simulink model "Electrical_System_2018b_obfs"  (R2019b)
settings: Solver=VariableStepAuto  StartTime=0.0  StopTime=5  RelTol=1e-3  AbsTol=1e-3  EnableMultiTasking=on
InitFcn:
  | Steady_State_Initialisation;
StopFcn:
  | %sscexplore(simlog);
  | %Logging
undefined symbols (not defined in the file): abrlhklxvp, aexgmhuedq, afmfmjnutg, afpphrjpnc, ahuxbyvruc, alarvljztt, amxnyqmnuw, aodrlwvqie, aolhmuplyq, aqpmguuqkg, auesgwirzl, aurophlnng, awamelrhru, ayfhvxflxn, azxkacuhqc, babszerikg, bawhdqanwq, bevoqecvei, bltjvqbchx, bmqsuewujl, bsmyqjfgnf, btvjbsmnve, bywgxqeadw, bziaduxaer, bzmcmdqocb, bzsvyvetat, ccsjnrbsih, cdvenygxwh, cedkrnslhx, cjheorclzs, cjrdshrtqx, ckhavyhcza, ckxewznhlz, cmrcgyiplk, conenicnws, cqkejbgjnn, csfnuwymhe, cunupkhwbh, cwzfvzuxxh, dcadmadufn, dcfponivnv, ddtrqjrhjn, dfhoxvkqas, dfrhtcwpne, dfvomcagjv, djijwylxea, dnmeqksrrm, dnzewbdkaa, dsqcykyxav, dtswwlttmm, ecumpidjtv, edegaywrct, ejjjsmnejc, eknqnehjdz, emvdetzouf, esxbqkbahr, etnkkbreiq, eunoiiiirw, ewewcuedir, fatkfxdhtc ... (+386)
libraries: fl_lib x802, ee_lib x362, fl_ps_legacy_lib x160, nesl_utility x85
(part 1 of 26)
settings Model: Creator=u617417  LastModifiedBy=u617417
settings SolverCC: AutoScaleAbsTol=off
settings DataIOCC: LimitDataPoints=on  MaxDataPoints=10000  ReturnWorkspaceOutputs=off
settings OptimizationCC: LifeSpan=inf
settings DebuggingCC: AllowSymbolicDim=off  SFUnexpectedBacktrackingDiag=warning  SFNoUnconditionalDefaultTransitionDiag=warning  SFExecutionAtInitializationDiag=none  ArithmeticOperatorsInVariantConditions=warning
settings SFSimCC: SimUseLocalCustomCode=off  CustomCodeUndefinedFunction=UseInterfaceOnly
settings RTWCC: RTWUseLocalCustomCode=off
settings CodeAppCC: StateflowObjectComments=on
settings GRTTargetCC: TargetLangStandard=C89/C90 (ANSI)  GeneratePreprocessorConditionals=Disable all
settings ConfigComp: CovMetricSettings=dw  CovHtmlReporting=on  CovSaveCumulativeToWorkspaceVar=on  CovSaveSingleToWorkspaceVar=on  CovExternalEMLEnable=off  CovSFcnEnable=off
settings SimscapeCC: SimscapeLogType=all  SimscapeLogDataHistory=10000

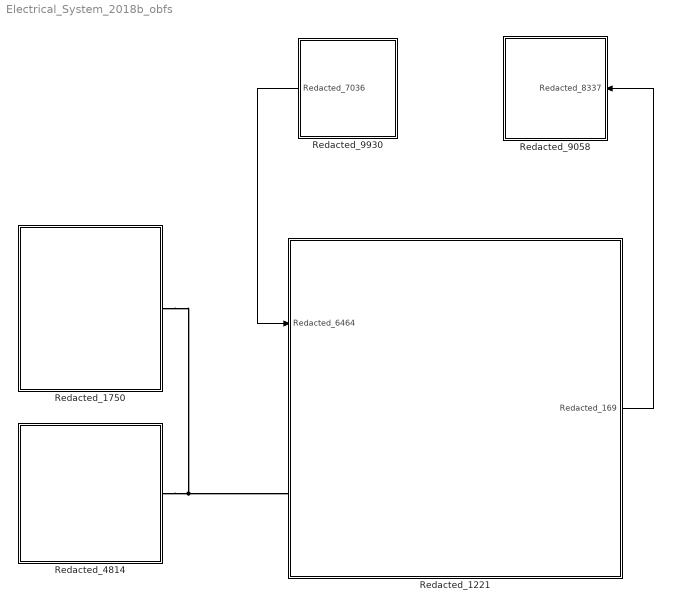
== system Electrical_System_2018b_obfs ==
  Redacted_1221 : Subsystem
  Redacted_1750 : Subsystem
  Redacted_4814 : Subsystem
  Redacted_9058 : Subsystem
  Redacted_9930 : Subsystem
  wires:
  Redacted_9930/1(Redacted_7036) -> Redacted_1221/1(Redacted_6464)
  Redacted_1221/1(Redacted_169) -> Redacted_9058/1(Redacted_8337)
  connections:
  Redacted_4814/RConn1 -- Redacted_1750/LConn1 -- Redacted_1221/LConn1

== system Electrical_System_2018b_obfs/Redacted_1221 ==
  Redacted_6464 : Inport
  Redacted_124 : BusCreator  Inputs=2
  Redacted_1290 : SimscapeBus  HierarchyStrings=Redacted_9542;Redacted_7385
  Redacted_346 : Subsystem
  Redacted_3922 : BusSelector  OutputSignals=Redacted1000,Redacted100
  Redacted_7523 : Subsystem
  Redacted_7580 : BusCreator  Inputs=2
  Redacted_7996 : Subsystem
  Redacted_7064 : PMIOPort  Side=Left
  Redacted_169 : Outport
  wires:
  Redacted_6464/1 -> Redacted_3922/1, Redacted_7996/1(Redacted_8884)
  Redacted_3922/2 -> Redacted_7523/1(Redacted_6806)  "<Redacted100>"
  Redacted_7996/1(Redacted_414) -> Redacted_7580/1
  Redacted_3922/1 -> Redacted_346/1(Redacted_388)  "<Redacted1000>"
  Redacted_124/1 -> Redacted_7580/2
  Redacted_7580/1 -> Redacted_169/1
  Redacted_346/1(Redacted_1936) -> Redacted_124/1
  Redacted_7523/1(Redacted_1117) -> Redacted_124/2
  connections:
  Redacted_7996/LConn1 -- Redacted_1290/RConn1 -- Redacted_7064/RConn1
  Redacted_7523/LConn1 -- Redacted_1290/LConn2
  Redacted_1290/LConn1 -- Redacted_346/LConn1

== system Electrical_System_2018b_obfs/Redacted_1750 ==
  Redacted_1744 : SimscapeBus  HierarchyStrings=Redacted_3580;Redacted_2679;Redacted_1356;Redacted_4546;Redacted_2723;Redacted_3875;Redacted_702;Redacted_7645;Redacted_1338;Redacted_3379;Redacted_7168;Redacted_7354;Redacted_1728;Redacted_6589;Redacted_3064;Redacted_7149;Redacted_7529;Redacted_4383;Redacted_4107;Redacted_3568;Redacted_6624;Redacted_6947;Redacted_2339;Redacted_4294;Redacted_5075;Redacted_5111;Redacted_7066;Redacted_1531;Redacted_7675;Redacted_9811;Redacted_5065;Redacted_4812;Redacted_9201;Redacted_6197;Redacted_8441;Redacted_5922;Redacted_720;Redacted_3478
  Redacted_1805 : SimscapeBus  HierarchyStrings=Redacted_9383;Redacted_6662
  Redacted_1925 : Subsystem  VariantControlMode=Label  Variant=on  VariantControl=Variant1  LabelModeActiveChoice=Choice
  Redacted_2252 : Subsystem  VariantControlMode=Label  Variant=on  VariantControl=Variant1  LabelModeActiveChoice=Choice
  Redacted_3116 : Subsystem  VariantControlMode=Label  Variant=on  VariantControl=Variant1  LabelModeActiveChoice=Variant1
  Redacted_342 : SimscapeBus  HierarchyStrings=Redacted_4753;Redacted_7074;Redacted_4542;Redacted_1072;Redacted_6392;Redacted_7262;Redacted_2302;Redacted_3799;Redacted_313;Redacted_3360;Redacted_9805;Redacted_7349;Redacted_7947;Redacted_2722;Redacted_9575;Redacted_197;Redacted_61;Redacted_5963;Redacted_4867;Redacted_743;Redacted_7386;Redacted_3425;Redacted_4607;Redacted_2034;Redacted_2575;Redacted_353;Redacted_234;Redacted_6669;Redacted_5669;Redacted_4890;Redacted_9806;Redacted_6181;Redacted_8668;Redacted_4306;Redacted_593;Redacted_8425;Redacted_5908;Redacted_8012;Redacted_3708;Redacted_3632;Redacted_250;Redacted_5917;Redacted_5879;Redacted_6182;Redacted_5408;Redacted_9552;Redacted_4609;Redacted_5680;Redacted_7438;Redacted_5551
  Redacted_3629 : Subsystem  VariantControlMode=Label  Variant=on  VariantControl=Variant1  LabelModeActiveChoice=Choice
  Redacted_3745 : SimscapeBus  HierarchyStrings=Redacted_1096;Redacted_3567
  Redacted_3761 : SimscapeBus  HierarchyStrings=Redacted_780;Redacted_28
  Redacted_393 : Subsystem  VariantControlMode=Label  Variant=on  VariantControl=Variant1  LabelModeActiveChoice=Choice
  Redacted_418 : Subsystem  VariantControlMode=Label  Variant=on  VariantControl=Variant1  LabelModeActiveChoice=Choice
  Redacted_4904 : nesl_utility/Solver Configuration  PhysicalDomain=network_engine_domain  SubClassName=solver  LeftPortType=input  RightPortType=generic  Tones=[]  Harmonics=[]  SimulateNoise=off  Profile=off  UseLocalSampling=off  EnableSwitchedLinearOptims=on  FrequencyDomain=off  UseCCode=off  RelTol=0.001  AbsTol=1e-06  MinStep=1e-09  ToWorkspace=off  RevertToSquareIcSolve=off  NumHomotopyIterations=100  PhasorMode=off  PhasorModeNumHarmonics=1  DoDC=on  ResidualTolerance=1e-09  UseLocalSolver=off  LocalSolverChoice=NE_BACKWARD_EULER_ADVANCER  LocalSolverSampleTime=0.001  DoFixedCost=off  MaxNonlinIter=3  MaxModeIter=2  LinearAlgebra=auto  EquationFormulation=NE_TIME_EF  DelaysMemoryBudget=1024  AutomaticFiltering=on  FilteringTimeConstant=0.001  PartitionStorageMethod=AS_NEEDED  PartitionMemoryBudget=1024  PartitionMethod=FAST
  Redacted_4947 : Subsystem
  Redacted_5338 : SimscapeBus  HierarchyStrings=Redacted_4565;Redacted_3565;Redacted_3754;Redacted_3229;Redacted_1463;Redacted_2424;Redacted_1593;Redacted_6398;Redacted_2122;Redacted_5759;Redacted_1474;Redacted_4040;Redacted_2796;Redacted_8639;Redacted_7131;Redacted_6318;Redacted_7850;Redacted_3335;Redacted_4313;Redacted_1636;Redacted_1179;Redacted_2852;Redacted_8529;Redacted_9943;Redacted_3136;Redacted_6249;Redacted_7332;Redacted_6303;Redacted_8216;Redacted_7695;Redacted_8718;Redacted_3072;Redacted_1178;Redacted_1890;Redacted_6383;Redacted_2665;Redacted_4351;Redacted_4540;Redacted_8937;Redacted_7401;Redacted_7023;Redacted_5287;Redacted_2225;Redacted_314;Redacted_4153;Redacted_6133;Redacted_6666;Redacted_1276;Redacted_2787;Redacted_6122
  Redacted_5639 : Subsystem
  Redacted_5682 : Subsystem  VariantControlMode=Label  Variant=on  VariantControl=Variant1  LabelModeActiveChoice=Choice
  Redacted_7456 : Subsystem  VariantControlMode=Label  Variant=on  VariantControl=Variant1  LabelModeActiveChoice=Variant1
  Redacted_7650 : Subsystem  VariantControlMode=Label  Variant=on  VariantControl=Variant1  LabelModeActiveChoice=Choice
  Redacted_8299 : Subsystem  VariantControlMode=Label  Variant=on  VariantControl=Variant1  LabelModeActiveChoice=Choice
  Redacted_8526 : SimscapeBus  HierarchyStrings=Redacted_5196;Redacted_4738;Redacted_9034;Redacted_8939;Redacted_5097;Redacted_5335;Redacted_8921;Redacted_9654;Redacted_7688;Redacted_4574;Redacted_6489;Redacted_3669;Redacted_1425;Redacted_9271;Redacted_8750;Redacted_5309;Redacted_2108;Redacted_3147;Redacted_7076;Redacted_768;Redacted_3463;Redacted_9121;Redacted_3800;Redacted_3593;Redacted_7030;Redacted_595;Redacted_9929;Redacted_1003;Redacted_3651;Redacted_3255;Redacted_1785;Redacted_2177;Redacted_6543;Redacted_5208;Redacted_247;Redacted_4433;Redacted_4655;Redacted_3962
  Redacted_8712 : Subsystem  VariantControlMode=Label  Variant=on  VariantControl=Variant1  LabelModeActiveChoice=Choice
  Redacted_1626 : PMIOPort  Side=Left
  connections:
  Redacted_418/LConn1 -- Redacted_342/LConn27
  Redacted_1744/LConn5 -- Redacted_4947/LConn5
  Redacted_418/LConn4 -- Redacted_342/LConn30
  Redacted_418/LConn3 -- Redacted_342/LConn29
  Redacted_1744/LConn1 -- Redacted_4947/LConn1
  Redacted_4947/LConn4 -- Redacted_1744/LConn4
  Redacted_1744/LConn3 -- Redacted_4947/LConn3
  Redacted_4947/LConn6 -- Redacted_1744/LConn6
  Redacted_418/LConn2 -- Redacted_342/LConn28
  Redacted_7650/LConn1 -- Redacted_342/LConn31
  Redacted_7650/LConn2 -- Redacted_342/LConn32
  Redacted_7650/LConn3 -- Redacted_342/LConn33
  Redacted_7650/LConn4 -- Redacted_342/LConn34
  Redacted_7650/LConn5 -- Redacted_342/LConn35
  Redacted_7650/LConn6 -- Redacted_342/LConn36
  Redacted_7650/LConn7 -- Redacted_342/LConn37
  Redacted_7650/LConn8 -- Redacted_342/LConn38
  Redacted_1925/LConn1 -- Redacted_342/LConn39
  Redacted_1925/LConn2 -- Redacted_342/LConn40
  Redacted_1925/LConn3 -- Redacted_342/LConn41
  Redacted_1925/LConn4 -- Redacted_342/LConn42
  Redacted_1925/LConn5 -- Redacted_342/LConn43
  Redacted_1925/LConn6 -- Redacted_342/LConn44
  Redacted_5338/LConn27 -- Redacted_393/LConn1
  Redacted_5338/LConn28 -- Redacted_393/LConn2
  Redacted_5338/LConn29 -- Redacted_393/LConn3
  Redacted_5338/LConn30 -- Redacted_393/LConn4
  Redacted_5338/LConn39 -- Redacted_8299/LConn1
  Redacted_5338/LConn40 -- Redacted_8299/LConn2
  Redacted_5338/LConn41 -- Redacted_8299/LConn3
  Redacted_5338/LConn42 -- Redacted_8299/LConn4
  Redacted_5338/LConn43 -- Redacted_8299/LConn5
  Redacted_5338/LConn44 -- Redacted_8299/LConn6
  Redacted_5338/LConn31 -- Redacted_3629/LConn1
  Redacted_5338/LConn32 -- Redacted_3629/LConn2
  Redacted_5338/LConn33 -- Redacted_3629/LConn3
  Redacted_5338/LConn34 -- Redacted_3629/LConn4
  Redacted_5338/LConn35 -- Redacted_3629/LConn5
  Redacted_5338/LConn36 -- Redacted_3629/LConn6
  Redacted_5338/LConn37 -- Redacted_3629/LConn7
  Redacted_5338/LConn38 -- Redacted_3629/LConn8
  Redacted_4904/RConn1 -- Redacted_5338/LConn47 -- Redacted_5682/RConn4
  Redacted_5682/LConn1 -- Redacted_342/LConn50
  Redacted_5682/LConn2 -- Redacted_342/LConn49
  Redacted_5682/LConn3 -- Redacted_342/LConn48
  Redacted_5682/LConn4 -- Redacted_342/LConn47
  Redacted_5338/LConn50 -- Redacted_5682/RConn1
  Redacted_5338/LConn49 -- Redacted_5682/RConn2
  Redacted_5338/LConn48 -- Redacted_5682/RConn3
  Redacted_4947/LConn2 -- Redacted_1744/LConn2
  Redacted_1744/LConn7 -- Redacted_4947/LConn7
  Redacted_4947/LConn8 -- Redacted_1744/LConn8
  Redacted_3745/RConn1 -- Redacted_1626/RConn1
  Redacted_1744/LConn9 -- Redacted_4947/LConn9
  Redacted_1744/LConn10 -- Redacted_4947/LConn10
  Redacted_1744/LConn14 -- Redacted_4947/LConn14
  Redacted_1744/LConn13 -- Redacted_4947/LConn13
  Redacted_1744/LConn12 -- Redacted_4947/LConn12
  Redacted_4947/LConn11 -- Redacted_1744/LConn11
  Redacted_1744/RConn1 -- Redacted_3761/LConn2
  Redacted_3761/LConn1 -- Redacted_342/RConn1
  Redacted_1805/LConn1 -- Redacted_5338/RConn1
  Redacted_3761/RConn1 -- Redacted_3745/LConn2
  Redacted_1805/RConn1 -- Redacted_3745/LConn1
  Redacted_4947/LConn15 -- Redacted_1744/LConn15
  Redacted_4947/LConn16 -- Redacted_1744/LConn16
  Redacted_4947/LConn17 -- Redacted_1744/LConn17
  Redacted_4947/LConn18 -- Redacted_1744/LConn18
  Redacted_4947/LConn19 -- Redacted_1744/LConn19
  Redacted_4947/LConn20 -- Redacted_1744/LConn20
  Redacted_4947/LConn21 -- Redacted_1744/LConn21
  Redacted_4947/LConn22 -- Redacted_1744/LConn22
  Redacted_4947/LConn23 -- Redacted_1744/LConn23
  Redacted_4947/LConn24 -- Redacted_1744/LConn24
  Redacted_4947/LConn25 -- Redacted_1744/LConn25
  Redacted_4947/LConn26 -- Redacted_1744/LConn26
  Redacted_4947/LConn27 -- Redacted_1744/LConn27
  Redacted_4947/LConn28 -- Redacted_1744/LConn28
  Redacted_4947/LConn29 -- Redacted_1744/LConn29
  Redacted_4947/LConn30 -- Redacted_1744/LConn30
  Redacted_2252/LConn1 -- Redacted_342/LConn1
  Redacted_2252/LConn2 -- Redacted_342/LConn2
  Redacted_2252/LConn3 -- Redacted_342/LConn3
  Redacted_2252/LConn4 -- Redacted_342/LConn4
  Redacted_2252/LConn5 -- Redacted_342/LConn5
  Redacted_2252/LConn6 -- Redacted_342/LConn6
  Redacted_2252/LConn7 -- Redacted_342/LConn7
  Redacted_2252/LConn8 -- Redacted_342/LConn8
  Redacted_2252/LConn9 -- Redacted_342/LConn9
  Redacted_2252/LConn10 -- Redacted_342/LConn10
  Redacted_2252/LConn11 -- Redacted_342/LConn11
  Redacted_2252/LConn12 -- Redacted_342/LConn12
  Redacted_2252/LConn13 -- Redacted_342/LConn13
  Redacted_2252/LConn14 -- Redacted_342/LConn14
  Redacted_2252/LConn15 -- Redacted_342/LConn15
  Redacted_2252/LConn16 -- Redacted_342/LConn16
  Redacted_2252/LConn17 -- Redacted_342/LConn17
  Redacted_2252/LConn18 -- Redacted_342/LConn18
  Redacted_2252/LConn19 -- Redacted_342/LConn19
  Redacted_2252/LConn20 -- Redacted_342/LConn20
  Redacted_2252/LConn21 -- Redacted_342/LConn21
  Redacted_2252/LConn22 -- Redacted_342/LConn22
  Redacted_2252/LConn23 -- Redacted_342/LConn23
  Redacted_2252/LConn24 -- Redacted_342/LConn24
  Redacted_2252/LConn25 -- Redacted_342/LConn25
  Redacted_2252/LConn26 -- Redacted_342/LConn26
  Redacted_4947/LConn31 -- Redacted_1744/LConn31
  Redacted_4947/LConn33 -- Redacted_1744/LConn33
  Redacted_4947/LConn35 -- Redacted_1744/LConn35
  Redacted_4947/LConn36 -- Redacted_1744/LConn36
  Redacted_4947/LConn37 -- Redacted_1744/LConn37
  Redacted_4947/LConn38 -- Redacted_1744/LConn38
  Redacted_4947/LConn34 -- Redacted_1744/LConn34
  Redacted_4947/LConn32 -- Redacted_1744/LConn32
  Redacted_8712/LConn1 -- Redacted_5338/LConn1
  Redacted_8712/LConn2 -- Redacted_5338/LConn2
  Redacted_8712/LConn3 -- Redacted_5338/LConn3
  Redacted_8712/LConn4 -- Redacted_5338/LConn4
  Redacted_8712/LConn5 -- Redacted_5338/LConn5
  Redacted_8712/LConn6 -- Redacted_5338/LConn6
  Redacted_8712/LConn7 -- Redacted_5338/LConn7
  Redacted_8712/LConn8 -- Redacted_5338/LConn8
  Redacted_8712/LConn9 -- Redacted_5338/LConn9
  Redacted_8712/LConn10 -- Redacted_5338/LConn10
  Redacted_8712/LConn11 -- Redacted_5338/LConn11
  Redacted_8712/LConn12 -- Redacted_5338/LConn12
  Redacted_8712/LConn13 -- Redacted_5338/LConn13
  Redacted_8712/LConn14 -- Redacted_5338/LConn14
  Redacted_8712/LConn15 -- Redacted_5338/LConn15
  Redacted_8712/LConn16 -- Redacted_5338/LConn16
  Redacted_8712/LConn17 -- Redacted_5338/LConn17
  Redacted_8712/LConn18 -- Redacted_5338/LConn18
  Redacted_8712/LConn19 -- Redacted_5338/LConn19
  Redacted_8712/LConn20 -- Redacted_5338/LConn20
  Redacted_8712/LConn21 -- Redacted_5338/LConn21
  Redacted_8712/LConn22 -- Redacted_5338/LConn22
  Redacted_8712/LConn23 -- Redacted_5338/LConn23
  Redacted_8712/LConn24 -- Redacted_5338/LConn24
  Redacted_8712/LConn25 -- Redacted_5338/LConn25
  Redacted_8712/LConn26 -- Redacted_5338/LConn26
  Redacted_5639/LConn32 -- Redacted_8526/LConn32
  Redacted_5639/LConn34 -- Redacted_8526/LConn34
  Redacted_5639/LConn37 -- Redacted_8526/LConn37
  Redacted_5639/LConn35 -- Redacted_8526/LConn35
  Redacted_5639/LConn33 -- Redacted_8526/LConn33
  Redacted_5639/LConn31 -- Redacted_8526/LConn31
  Redacted_5639/LConn30 -- Redacted_8526/LConn30
  Redacted_5639/LConn29 -- Redacted_8526/LConn29
  Redacted_5639/LConn28 -- Redacted_8526/LConn28
  Redacted_5639/LConn36 -- Redacted_8526/LConn36
  Redacted_5639/LConn27 -- Redacted_8526/LConn27
  Redacted_5639/LConn25 -- Redacted_8526/LConn25
  Redacted_5639/LConn24 -- Redacted_8526/LConn24
  Redacted_5639/LConn23 -- Redacted_8526/LConn23
  Redacted_5639/LConn22 -- Redacted_8526/LConn22
  Redacted_5639/LConn21 -- Redacted_8526/LConn21
  Redacted_5639/LConn20 -- Redacted_8526/LConn20
  Redacted_5639/LConn19 -- Redacted_8526/LConn19
  Redacted_5639/LConn18 -- Redacted_8526/LConn18
  Redacted_5639/LConn17 -- Redacted_8526/LConn17
  Redacted_5639/LConn16 -- Redacted_8526/LConn16
  Redacted_5639/LConn26 -- Redacted_8526/LConn26
  Redacted_5639/LConn38 -- Redacted_8526/LConn38
  Redacted_5639/LConn15 -- Redacted_8526/LConn15
  Redacted_5639/LConn11 -- Redacted_8526/LConn11
  Redacted_8526/LConn12 -- Redacted_5639/LConn12
  Redacted_8526/LConn13 -- Redacted_5639/LConn13
  Redacted_8526/LConn10 -- Redacted_5639/LConn10
  Redacted_8526/LConn9 -- Redacted_5639/LConn9
  Redacted_5639/LConn8 -- Redacted_8526/LConn8
  Redacted_5639/LConn6 -- Redacted_8526/LConn6
  Redacted_8526/LConn7 -- Redacted_5639/LConn7
  Redacted_8526/LConn3 -- Redacted_5639/LConn3
  Redacted_5639/LConn4 -- Redacted_8526/LConn4
  Redacted_8526/LConn1 -- Redacted_5639/LConn1
  Redacted_8526/LConn14 -- Redacted_5639/LConn14
  Redacted_8526/LConn5 -- Redacted_5639/LConn5
  Redacted_5639/LConn2 -- Redacted_8526/LConn2
  Redacted_8526/RConn1 -- Redacted_1805/LConn2
  Redacted_3116/LConn1 -- Redacted_342/LConn45
  Redacted_3116/LConn2 -- Redacted_342/LConn46
  Redacted_7456/LConn1 -- Redacted_5338/LConn45
  Redacted_7456/LConn2 -- Redacted_5338/LConn46

== system Electrical_System_2018b_obfs/Redacted_4814 ==
  Redacted_1188 : SimscapeBus  HierarchyStrings=Redacted_5170;Redacted_3456
  Redacted_1224 : SimscapeBus  HierarchyStrings=Redacted_5417;Redacted_5050
  Redacted_1389 : SimscapeBus  HierarchyStrings=Redacted_4470;Redacted_2451
  Redacted_3297 : Subsystem  VariantControlMode=Label  Variant=on  VariantControl=Variant1  LabelModeActiveChoice=Choice
  Redacted_3902 : SimscapeBus  HierarchyStrings=Redacted_1356;Redacted_9036
  Redacted_3928 : Subsystem  VariantControlMode=Label  Variant=on  VariantControl=Variant1  LabelModeActiveChoice=Choice
  Redacted_7520 : SimscapeBus  HierarchyStrings=Redacted_3429;Redacted_1098
  Redacted_8098 : SimscapeBus  HierarchyStrings=Redacted_379;Redacted_2486
  Redacted_8799 : SimscapeBus  HierarchyStrings=Redacted_3276;Redacted_5658
  Redacted_9979 : PMIOPort  Side=Right
  connections:
  Redacted_3297/RConn1 -- Redacted_8098/LConn1
  Redacted_1188/RConn1 -- Redacted_9979/RConn1
  Redacted_7520/RConn1 -- Redacted_1188/LConn2
  Redacted_8098/LConn2 -- Redacted_3297/RConn2
  Redacted_8799/LConn2 -- Redacted_3297/RConn4
  Redacted_8799/LConn1 -- Redacted_3297/RConn3
  Redacted_1389/LConn2 -- Redacted_8799/RConn1
  Redacted_1389/LConn1 -- Redacted_8098/RConn1
  Redacted_1389/RConn1 -- Redacted_1188/LConn1
  Redacted_7520/LConn1 -- Redacted_3902/RConn1
  Redacted_7520/LConn2 -- Redacted_1224/RConn1
  Redacted_3902/LConn1 -- Redacted_3928/RConn1
  Redacted_3902/LConn2 -- Redacted_3928/RConn2
  Redacted_3928/RConn3 -- Redacted_1224/LConn1
  Redacted_3928/RConn4 -- Redacted_1224/LConn2

== system Electrical_System_2018b_obfs/Redacted_9058 ==
  Redacted_8337 : Inport
  Redacted_8297 : Terminator
  wires:
  Redacted_8337/1 -> Redacted_8297/1

== system Electrical_System_2018b_obfs/Redacted_9930 ==
  Redacted_2381 : BusCreator  Inputs=30
  Redacted_3896 : Subsystem  VariantControlMode=Label  Variant=on  VariantControl=Variant1  LabelModeActiveChoice=Variant1
  Redacted_4112 : BusCreator  Inputs=30
  Redacted_4814 : Subsystem  VariantControlMode=Label  Variant=on  VariantControl=Variant1  LabelModeActiveChoice=Variant1
  Redacted_6072 : BusCreator  Inputs=2
  Redacted_7036 : Outport
  wires:
  Redacted_6072/1 -> Redacted_7036/1
  Redacted_4112/1 -> Redacted_6072/2  "Redacted1000"
  Redacted_2381/1 -> Redacted_6072/1  "Redacted100"
  Redacted_3896/1(Redacted_644) -> Redacted_2381/1
  Redacted_3896/2(Redacted_2723) -> Redacted_2381/2
  Redacted_3896/3(Redacted_8075) -> Redacted_2381/3
  Redacted_3896/4(Redacted_4126) -> Redacted_2381/4
  Redacted_3896/5(Redacted_7964) -> Redacted_2381/5
  Redacted_3896/6(Redacted_8682) -> Redacted_2381/6
  Redacted_3896/7(Redacted_6320) -> Redacted_2381/7
  Redacted_3896/8(Redacted_340) -> Redacted_2381/8
  Redacted_3896/9(Redacted_2756) -> Redacted_2381/9
  Redacted_3896/10(Redacted_3273) -> Redacted_2381/10
  Redacted_3896/11(Redacted_4657) -> Redacted_2381/11
  Redacted_3896/12(Redacted_3395) -> Redacted_2381/12
  Redacted_3896/13(Redacted_9977) -> Redacted_2381/13
  Redacted_3896/14(Redacted_2599) -> Redacted_2381/14
  Redacted_3896/15(Redacted_1407) -> Redacted_2381/15
  Redacted_3896/16(Redacted_9412) -> Redacted_2381/16
  Redacted_3896/17(Redacted_123) -> Redacted_2381/17
  Redacted_3896/18(Redacted_8209) -> Redacted_2381/18
  Redacted_3896/19(Redacted_531) -> Redacted_2381/19
  Redacted_3896/20(Redacted_6389) -> Redacted_2381/20
  Redacted_3896/21(Redacted_6836) -> Redacted_2381/21
  Redacted_3896/22(Redacted_5007) -> Redacted_2381/22
  Redacted_3896/23(Redacted_6497) -> Redacted_2381/23
  Redacted_3896/24(Redacted_9632) -> Redacted_2381/24
  Redacted_3896/25(Redacted_2902) -> Redacted_2381/25
  Redacted_3896/26(Redacted_2695) -> Redacted_2381/26
  Redacted_3896/27(Redacted_8396) -> Redacted_2381/27
  Redacted_3896/28(Redacted_9164) -> Redacted_2381/28
  Redacted_3896/29(Redacted_9075) -> Redacted_2381/29
  Redacted_3896/30(Redacted_6090) -> Redacted_2381/30
  Redacted_4814/1(Redacted_6479) -> Redacted_4112/1
  Redacted_4814/2(Redacted_3532) -> Redacted_4112/2
  Redacted_4814/3(Redacted_6579) -> Redacted_4112/3
  Redacted_4814/4(Redacted_5091) -> Redacted_4112/4
  Redacted_4814/5(Redacted_5066) -> Redacted_4112/5
  Redacted_4814/6(Redacted_2648) -> Redacted_4112/6
  Redacted_4814/7(Redacted_3799) -> Redacted_4112/7
  Redacted_4814/8(Redacted_988) -> Redacted_4112/8
  Redacted_4814/9(Redacted_4741) -> Redacted_4112/9
  Redacted_4814/10(Redacted_474) -> Redacted_4112/10
  Redacted_4814/11(Redacted_4041) -> Redacted_4112/11
  Redacted_4814/12(Redacted_9998) -> Redacted_4112/12
  Redacted_4814/13(Redacted_2742) -> Redacted_4112/13
  Redacted_4814/14(Redacted_5781) -> Redacted_4112/14
  Redacted_4814/15(Redacted_125) -> Redacted_4112/15
  Redacted_4814/16(Redacted_4308) -> Redacted_4112/16
  Redacted_4814/17(Redacted_8077) -> Redacted_4112/17
  Redacted_4814/18(Redacted_7701) -> Redacted_4112/18
  Redacted_4814/19(Redacted_8967) -> Redacted_4112/19
  Redacted_4814/20(Redacted_8464) -> Redacted_4112/20
  Redacted_4814/21(Redacted_1093) -> Redacted_4112/21
  Redacted_4814/22(Redacted_1950) -> Redacted_4112/22
  Redacted_4814/23(Redacted_1167) -> Redacted_4112/23
  Redacted_4814/24(Redacted_3969) -> Redacted_4112/24
  Redacted_4814/25(Redacted_1905) -> Redacted_4112/25
  Redacted_4814/26(Redacted_1688) -> Redacted_4112/26
  Redacted_4814/27(Redacted_6009) -> Redacted_4112/27
  Redacted_4814/28(Redacted_9612) -> Redacted_4112/28
  Redacted_4814/29(Redacted_8082) -> Redacted_4112/29
  Redacted_4814/30(Redacted_1556) -> Redacted_4112/30

== system Electrical_System_2018b_obfs/Redacted_1221/Redacted_346 ==
  Redacted_388 : Inport
  Redacted_2722 : Subsystem
  Redacted_2760 : BusCreator  Inputs=4
  Redacted_3067 : Subsystem
  Redacted_5295 : Subsystem
  Redacted_6610 : Subsystem
  Redacted_3749 : PMIOPort  Side=Left
  Redacted_1936 : Outport
  wires:
  Redacted_388/1 -> Redacted_5295/1(Redacted_8545), Redacted_2722/1(Redacted_6167), Redacted_3067/1(Redacted_882), Redacted_6610/1(Redacted_3546)
  Redacted_5295/1(Redacted_7641) -> Redacted_2760/1
  Redacted_2760/1 -> Redacted_1936/1
  Redacted_6610/1(Redacted_1746) -> Redacted_2760/2
  Redacted_3067/1(Redacted_7765) -> Redacted_2760/3
  Redacted_2722/1(Redacted_1476) -> Redacted_2760/4
  connections:
  Redacted_5295/LConn1 -- Redacted_3749/RConn1 -- Redacted_6610/LConn1 -- Redacted_3067/LConn1 -- Redacted_2722/LConn1

== system Electrical_System_2018b_obfs/Redacted_1221/Redacted_7523 ==
  Redacted_6806 : Inport
  Redacted_1100 : BusCreator  Inputs=4
  Redacted_2432 : Subsystem
  Redacted_5456 : Subsystem
  Redacted_5495 : Subsystem
  Redacted_6578 : Subsystem
  Redacted_332 : PMIOPort  Side=Left
  Redacted_1117 : Outport
  wires:
  Redacted_6806/1 -> Redacted_5456/1(Redacted_8021), Redacted_6578/1(Redacted_753), Redacted_2432/1(Redacted_3217), Redacted_5495/1(Redacted_4129)
  Redacted_5456/1(Redacted_3690) -> Redacted_1100/1
  Redacted_1100/1 -> Redacted_1117/1
  Redacted_5495/1(Redacted_3176) -> Redacted_1100/2
  Redacted_2432/1(Redacted_9205) -> Redacted_1100/3
  Redacted_6578/1(Redacted_9705) -> Redacted_1100/4
  connections:
  Redacted_5456/LConn1 -- Redacted_332/RConn1 -- Redacted_5495/LConn1 -- Redacted_2432/LConn1 -- Redacted_6578/LConn1

== system Electrical_System_2018b_obfs/Redacted_1221/Redacted_7996 ==
  Redacted_8884 : Inport
  Redacted_1 : Subsystem
  Redacted_124 : BusCreator  Inputs=4
  Redacted_1427 : fl_lib/Electrical/Electrical Elements/Resistor  R=izkxgsjeum Ohm  i_specify=off  i_priority=None  i=okctexlfdc A  i_nominal_specify=off  i_nominal_unit=A  i_nominal_value=krtyyeteoe  v_specify=off  v_priority=None  v=jsorwthgpb V  v_nominal_specify=off  v_nominal_unit=V  v_nominal_value=vlyvqyoeya
  Redacted_2 : Subsystem
  Redacted_3272 : SimscapeBus  HierarchyStrings=Redacted_7407;Redacted_4715
  Redacted_5057 : fl_lib/Electrical/Electrical Elements/Electrical Reference
  Redacted_5406 : BusSelector  OutputSignals=Redacted100,Redacted1000
  Redacted_7418 : Subsystem
  Redacted_9242 : Subsystem
  Redacted_2185 : PMIOPort  Side=Left
  Redacted_414 : Outport
  wires:
  Redacted_5406/2 -> Redacted_9242/1(Redacted_9139), Redacted_7418/1(Redacted_5759)  "<Redacted1000>"
  Redacted_8884/1 -> Redacted_5406/1
  Redacted_5406/1 -> Redacted_1/1(Redacted_5759), Redacted_2/1(Redacted_9139)  "<Redacted100>"
  Redacted_9242/1(Redacted_9750) -> Redacted_124/2
  Redacted_124/1 -> Redacted_414/1
  Redacted_7418/1(Redacted_4777) -> Redacted_124/1
  Redacted_1/1(Redacted_4777) -> Redacted_124/3
  Redacted_2/1(Redacted_9750) -> Redacted_124/4
  connections:
  Redacted_3272/RConn1 -- Redacted_2185/RConn1
  Redacted_5057/LConn1 -- Redacted_1427/RConn1
  Redacted_9242/RConn3 -- Redacted_7418/RConn1
  Redacted_7418/RConn2 -- Redacted_9242/RConn2
  Redacted_7418/RConn3 -- Redacted_9242/RConn1
  Redacted_1/RConn3 -- Redacted_2/RConn1
  Redacted_1/RConn2 -- Redacted_2/RConn2
  Redacted_1/RConn1 -- Redacted_2/RConn3
  Redacted_2/RConn4 -- Redacted_9242/RConn4
  Redacted_2/RConn6 -- Redacted_9242/RConn6
  Redacted_1427/LConn1 -- Redacted_2/RConn5 -- Redacted_9242/RConn5
  Redacted_9242/LConn1 -- Redacted_7418/LConn1 -- Redacted_3272/LConn2
  Redacted_3272/LConn1 -- Redacted_1/LConn1 -- Redacted_2/LConn1

== system Electrical_System_2018b_obfs/Redacted_1750/Redacted_1925 ==
  note: Steady State
  note: Transient
  Redacted_8189 : Subsystem  VariantControl=Choice
  Redacted_191 : PMIOPort  Side=Left
  Redacted_5684 : PMIOPort  Port=2  Side=Left
  Redacted_8638 : PMIOPort  Port=3  Side=Left
  Redacted_2799 : PMIOPort  Port=4  Side=Left
  Redacted_4825 : PMIOPort  Port=5  Side=Left
  Redacted_997 : PMIOPort  Port=6  Side=Left

== system Electrical_System_2018b_obfs/Redacted_1750/Redacted_2252 ==
  note: Transient
  note: Steady State
  Redacted_5114 : Subsystem  VariantControl=Choice
  Redacted_8300 : PMIOPort  Side=Left
  Redacted_50 : PMIOPort  Port=2  Side=Left
  Redacted_1513 : PMIOPort  Port=3  Side=Left
  Redacted_4142 : PMIOPort  Port=4  Side=Left
  Redacted_9072 : PMIOPort  Port=5  Side=Left
  Redacted_8330 : PMIOPort  Port=6  Side=Left
  Redacted_1895 : PMIOPort  Port=7  Side=Left
  Redacted_7870 : PMIOPort  Port=8  Side=Left
  Redacted_4399 : PMIOPort  Port=9  Side=Left
  Redacted_3718 : PMIOPort  Port=10  Side=Left
  Redacted_5529 : PMIOPort  Port=11  Side=Left
  Redacted_1897 : PMIOPort  Port=12  Side=Left
  Redacted_5095 : PMIOPort  Port=13  Side=Left
  Redacted_5373 : PMIOPort  Port=14  Side=Left
  Redacted_7138 : PMIOPort  Port=15  Side=Left
  Redacted_444 : PMIOPort  Port=16  Side=Left
  Redacted_105 : PMIOPort  Port=17  Side=Left
  Redacted_9052 : PMIOPort  Port=18  Side=Left
  Redacted_7634 : PMIOPort  Port=19  Side=Left
  Redacted_7555 : PMIOPort  Port=20  Side=Left
  Redacted_6684 : PMIOPort  Port=21  Side=Left
  Redacted_7517 : PMIOPort  Port=22  Side=Left
  Redacted_9903 : PMIOPort  Port=23  Side=Left
  Redacted_4196 : PMIOPort  Port=24  Side=Left
  Redacted_7593 : PMIOPort  Port=25  Side=Left
  Redacted_5814 : PMIOPort  Port=26  Side=Left

== system Electrical_System_2018b_obfs/Redacted_1750/Redacted_3116 ==
  note: Transient
  note: Steady State
  Redacted_9404 : Subsystem  VariantControl=Variant1
  Redacted_6078 : PMIOPort  Side=Left
  Redacted_7382 : PMIOPort  Port=2  Side=Left

== system Electrical_System_2018b_obfs/Redacted_1750/Redacted_3629 ==
  note: Transient
  note: Steady State
  Redacted_3983 : Subsystem  VariantControl=Choice
  Redacted_6800 : PMIOPort  Side=Left
  Redacted_9542 : PMIOPort  Port=2  Side=Left
  Redacted_69 : PMIOPort  Port=3  Side=Left
  Redacted_2733 : PMIOPort  Port=4  Side=Left
  Redacted_3154 : PMIOPort  Port=5  Side=Left
  Redacted_8226 : PMIOPort  Port=6  Side=Left
  Redacted_2945 : PMIOPort  Port=7  Side=Left
  Redacted_9173 : PMIOPort  Port=8  Side=Left

== system Electrical_System_2018b_obfs/Redacted_1750/Redacted_393 ==
  note: Steady State
  note: Transient
  Redacted_3640 : Subsystem  VariantControl=Choice
  Redacted_8912 : PMIOPort  Side=Left
  Redacted_9942 : PMIOPort  Port=2  Side=Left
  Redacted_6824 : PMIOPort  Port=3  Side=Left
  Redacted_5238 : PMIOPort  Port=4  Side=Left

== system Electrical_System_2018b_obfs/Redacted_1750/Redacted_418 ==
  note: Transient
  note: Steady State
  Redacted_6987 : Subsystem  VariantControl=Choice
  Redacted_1593 : PMIOPort  Side=Left
  Redacted_8573 : PMIOPort  Port=2  Side=Left
  Redacted_2123 : PMIOPort  Port=3  Side=Left
  Redacted_5119 : PMIOPort  Port=4  Side=Left

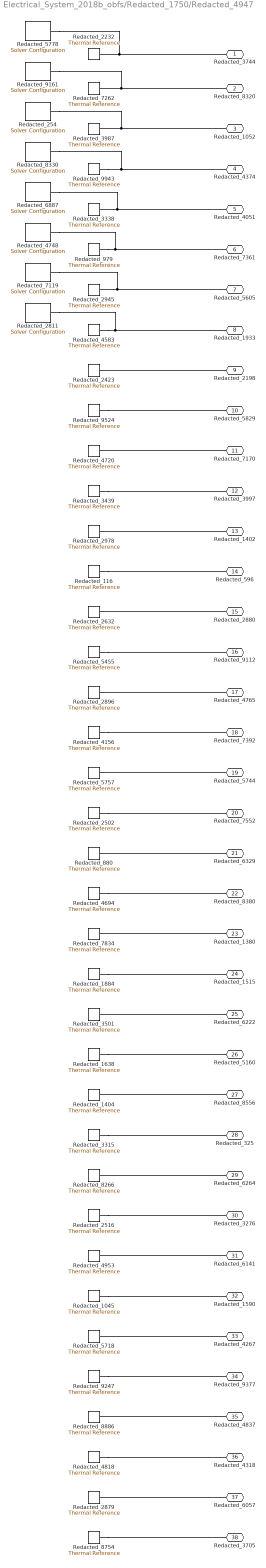
== system Electrical_System_2018b_obfs/Redacted_1750/Redacted_4947 ==
  Redacted_{116,880,979,1045,1404,1638,1884,2232,2423,2502,2516,2632,2879,2896,2945,2978,3315,3338,3439,3501,3987,4156,4583,4694,4720,4818,4953,5455,5718,5757,7262,7834,8266,8754,8886,9247,9524,9943} (38 alike) : fl_lib/Thermal/Thermal Elements/Thermal Reference
  Redacted_{254,2811,4748,5778,6887,7119,8330,9161} (8 alike) : nesl_utility/Solver Configuration  PhysicalDomain=network_engine_domain  SubClassName=solver  LeftPortType=input  RightPortType=generic  Tones=[]  Harmonics=[]  SimulateNoise=off  Profile=off  UseLocalSampling=off  EnableSwitchedLinearOptims=on  FrequencyDomain=off  UseCCode=off  RelTol=0.001  AbsTol=1e-06  MinStep=1e-09  ToWorkspace=off  RevertToSquareIcSolve=off  NumHomotopyIterations=100  PhasorMode=off  PhasorModeNumHarmonics=1  DoDC=off  ResidualTolerance=1e-09  UseLocalSolver=off  LocalSolverChoice=NE_BACKWARD_EULER_ADVANCER  LocalSolverSampleTime=0.001  DoFixedCost=off  MaxNonlinIter=3  MaxModeIter=2  LinearAlgebra=auto  EquationFormulation=NE_TIME_EF  DelaysMemoryBudget=1024  AutomaticFiltering=on  FilteringTimeConstant=0.001  PartitionStorageMethod=AS_NEEDED  PartitionMemoryBudget=1024  PartitionMethod=ROBUST
  Redacted_3744 : PMIOPort  Side=Left
  Redacted_8320 : PMIOPort  Port=2  Side=Left
  Redacted_1052 : PMIOPort  Port=3  Side=Left
  Redacted_4374 : PMIOPort  Port=4  Side=Left
  Redacted_4051 : PMIOPort  Port=5  Side=Left
  Redacted_7361 : PMIOPort  Port=6  Side=Left
  Redacted_5605 : PMIOPort  Port=7  Side=Left
  Redacted_1933 : PMIOPort  Port=8  Side=Left
  Redacted_2198 : PMIOPort  Port=9  Side=Left
  Redacted_5829 : PMIOPort  Port=10  Side=Left
  Redacted_7170 : PMIOPort  Port=11  Side=Left
  Redacted_3997 : PMIOPort  Port=12  Side=Left
  Redacted_1402 : PMIOPort  Port=13  Side=Left
  Redacted_596 : PMIOPort  Port=14  Side=Left
  Redacted_2880 : PMIOPort  Port=15  Side=Left
  Redacted_9112 : PMIOPort  Port=16  Side=Left
  Redacted_4765 : PMIOPort  Port=17  Side=Left
  Redacted_7392 : PMIOPort  Port=18  Side=Left
  Redacted_5744 : PMIOPort  Port=19  Side=Left
  Redacted_7552 : PMIOPort  Port=20  Side=Left
  Redacted_6329 : PMIOPort  Port=21  Side=Left
  Redacted_8380 : PMIOPort  Port=22  Side=Left
  Redacted_1380 : PMIOPort  Port=23  Side=Left
  Redacted_1515 : PMIOPort  Port=24  Side=Left
  Redacted_6222 : PMIOPort  Port=25  Side=Left
  Redacted_5160 : PMIOPort  Port=26  Side=Left
  Redacted_8556 : PMIOPort  Port=27  Side=Left
  Redacted_325 : PMIOPort  Port=28  Side=Left
  Redacted_6264 : PMIOPort  Port=29  Side=Left
  Redacted_3276 : PMIOPort  Port=30  Side=Left
  Redacted_6141 : PMIOPort  Port=31  Side=Left
  Redacted_1590 : PMIOPort  Port=32  Side=Left
  Redacted_4267 : PMIOPort  Port=33  Side=Left
  Redacted_9377 : PMIOPort  Port=34  Side=Left
  Redacted_4837 : PMIOPort  Port=35  Side=Left
  Redacted_4318 : PMIOPort  Port=36  Side=Left
  Redacted_6057 : PMIOPort  Port=37  Side=Left
  Redacted_3705 : PMIOPort  Port=38  Side=Left
  connections:
  Redacted_3744/RConn1 -- Redacted_5778/RConn1 -- Redacted_2232/LConn1
  Redacted_4051/RConn1 -- Redacted_6887/RConn1 -- Redacted_3338/LConn1
  Redacted_9943/LConn1 -- Redacted_8330/RConn1 -- Redacted_4374/RConn1
  Redacted_1052/RConn1 -- Redacted_254/RConn1 -- Redacted_3987/LConn1
  Redacted_979/LConn1 -- Redacted_4748/RConn1 -- Redacted_7361/RConn1
  Redacted_8320/RConn1 -- Redacted_9161/RConn1 -- Redacted_7262/LConn1
  Redacted_5605/RConn1 -- Redacted_2945/LConn1 -- Redacted_7119/RConn1
  Redacted_4583/LConn1 -- Redacted_1933/RConn1 -- Redacted_2811/RConn1
  Redacted_1402/RConn1 -- Redacted_2978/LConn1
  Redacted_2198/RConn1 -- Redacted_2423/LConn1
  Redacted_116/LConn1 -- Redacted_596/RConn1
  Redacted_9524/LConn1 -- Redacted_5829/RConn1
  Redacted_3439/LConn1 -- Redacted_3997/RConn1
  Redacted_7170/RConn1 -- Redacted_4720/LConn1
  Redacted_4156/LConn1 -- Redacted_7392/RConn1
  Redacted_4765/RConn1 -- Redacted_2896/LConn1
  Redacted_5455/LConn1 -- Redacted_9112/RConn1
  Redacted_2502/LConn1 -- Redacted_7552/RConn1
  Redacted_2880/RConn1 -- Redacted_2632/LConn1
  Redacted_5744/RConn1 -- Redacted_5757/LConn1
  Redacted_6222/RConn1 -- Redacted_3501/LConn1
  Redacted_1638/LConn1 -- Redacted_5160/RConn1
  Redacted_4694/LConn1 -- Redacted_8380/RConn1
  Redacted_6329/RConn1 -- Redacted_880/LConn1
  Redacted_1380/RConn1 -- Redacted_7834/LConn1
  Redacted_1884/LConn1 -- Redacted_1515/RConn1
  Redacted_6264/RConn1 -- Redacted_8266/LConn1
  Redacted_8556/RConn1 -- Redacted_1404/LConn1
  Redacted_3315/LConn1 -- Redacted_325/RConn1
  Redacted_2516/LConn1 -- Redacted_3276/RConn1
  Redacted_6057/RConn1 -- Redacted_2879/LConn1
  Redacted_6141/RConn1 -- Redacted_4953/LConn1
  Redacted_4818/LConn1 -- Redacted_4318/RConn1
  Redacted_9247/LConn1 -- Redacted_9377/RConn1
  Redacted_1045/LConn1 -- Redacted_1590/RConn1
  Redacted_4837/RConn1 -- Redacted_8886/LConn1
  Redacted_4267/RConn1 -- Redacted_5718/LConn1
  Redacted_8754/LConn1 -- Redacted_3705/RConn1

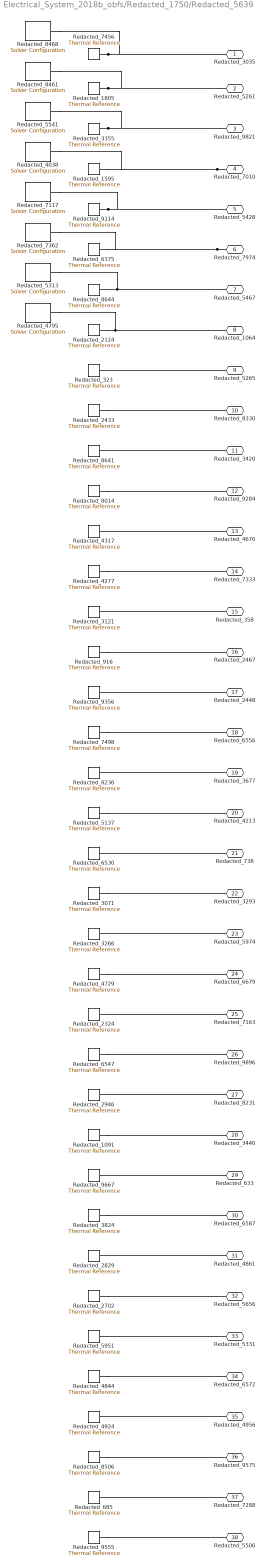
== system Electrical_System_2018b_obfs/Redacted_1750/Redacted_5639 ==
  Redacted_{323,685,916,1091,1595,1805,2124,2324,2433,2702,2829,2946,3071,3121,3266,3355,3824,4277,4317,4729,4844,4924,5137,5951,6375,6530,6547,7456,7498,8014,8236,8506,8641,8644,9114,9356,9555,9667} (38 alike) : fl_lib/Thermal/Thermal Elements/Thermal Reference
  Redacted_{4038,4795,5313,5541,7117,7362,8461,8468} (8 alike) : nesl_utility/Solver Configuration  PhysicalDomain=network_engine_domain  SubClassName=solver  LeftPortType=input  RightPortType=generic  Tones=[]  Harmonics=[]  SimulateNoise=off  Profile=off  UseLocalSampling=off  EnableSwitchedLinearOptims=on  FrequencyDomain=off  UseCCode=off  RelTol=0.001  AbsTol=1e-06  MinStep=1e-09  ToWorkspace=off  RevertToSquareIcSolve=off  NumHomotopyIterations=100  PhasorMode=off  PhasorModeNumHarmonics=1  DoDC=off  ResidualTolerance=1e-09  UseLocalSolver=off  LocalSolverChoice=NE_BACKWARD_EULER_ADVANCER  LocalSolverSampleTime=0.001  DoFixedCost=off  MaxNonlinIter=3  MaxModeIter=2  LinearAlgebra=auto  EquationFormulation=NE_TIME_EF  DelaysMemoryBudget=1024  AutomaticFiltering=on  FilteringTimeConstant=0.001  PartitionStorageMethod=AS_NEEDED  PartitionMemoryBudget=1024  PartitionMethod=ROBUST
  Redacted_3035 : PMIOPort  Side=Left
  Redacted_5261 : PMIOPort  Port=2  Side=Left
  Redacted_9821 : PMIOPort  Port=3  Side=Left
  Redacted_7010 : PMIOPort  Port=4  Side=Left
  Redacted_5428 : PMIOPort  Port=5  Side=Left
  Redacted_7974 : PMIOPort  Port=6  Side=Left
  Redacted_5467 : PMIOPort  Port=7  Side=Left
  Redacted_1064 : PMIOPort  Port=8  Side=Left
  Redacted_5265 : PMIOPort  Port=9  Side=Left
  Redacted_8330 : PMIOPort  Port=10  Side=Left
  Redacted_3420 : PMIOPort  Port=11  Side=Left
  Redacted_9284 : PMIOPort  Port=12  Side=Left
  Redacted_4670 : PMIOPort  Port=13  Side=Left
  Redacted_7333 : PMIOPort  Port=14  Side=Left
  Redacted_358 : PMIOPort  Port=15  Side=Left
  Redacted_2467 : PMIOPort  Port=16  Side=Left
  Redacted_2448 : PMIOPort  Port=17  Side=Left
  Redacted_6556 : PMIOPort  Port=18  Side=Left
  Redacted_3677 : PMIOPort  Port=19  Side=Left
  Redacted_4213 : PMIOPort  Port=20  Side=Left
  Redacted_738 : PMIOPort  Port=21  Side=Left
  Redacted_3293 : PMIOPort  Port=22  Side=Left
  Redacted_5974 : PMIOPort  Port=23  Side=Left
  Redacted_6679 : PMIOPort  Port=24  Side=Left
  Redacted_7163 : PMIOPort  Port=25  Side=Left
  Redacted_9896 : PMIOPort  Port=26  Side=Left
  Redacted_8231 : PMIOPort  Port=27  Side=Left
  Redacted_3440 : PMIOPort  Port=28  Side=Left
  Redacted_633 : PMIOPort  Port=29  Side=Left
  Redacted_6587 : PMIOPort  Port=30  Side=Left
  Redacted_4861 : PMIOPort  Port=31  Side=Left
  Redacted_5656 : PMIOPort  Port=32  Side=Left
  Redacted_5331 : PMIOPort  Port=33  Side=Left
  Redacted_6572 : PMIOPort  Port=34  Side=Left
  Redacted_4956 : PMIOPort  Port=35  Side=Left
  Redacted_9575 : PMIOPort  Port=36  Side=Left
  Redacted_7288 : PMIOPort  Port=37  Side=Left
  Redacted_5506 : PMIOPort  Port=38  Side=Left
  connections:
  Redacted_9555/LConn1 -- Redacted_5506/RConn1
  Redacted_5331/RConn1 -- Redacted_5951/LConn1
  Redacted_4956/RConn1 -- Redacted_4924/LConn1
  Redacted_2702/LConn1 -- Redacted_5656/RConn1
  Redacted_4844/LConn1 -- Redacted_6572/RConn1
  Redacted_8506/LConn1 -- Redacted_9575/RConn1
  Redacted_4861/RConn1 -- Redacted_2829/LConn1
  Redacted_7288/RConn1 -- Redacted_685/LConn1
  Redacted_3824/LConn1 -- Redacted_6587/RConn1
  Redacted_1091/LConn1 -- Redacted_3440/RConn1
  Redacted_8231/RConn1 -- Redacted_2946/LConn1
  Redacted_633/RConn1 -- Redacted_9667/LConn1
  Redacted_4729/LConn1 -- Redacted_6679/RConn1
  Redacted_5974/RConn1 -- Redacted_3266/LConn1
  Redacted_738/RConn1 -- Redacted_6530/LConn1
  Redacted_3071/LConn1 -- Redacted_3293/RConn1
  Redacted_6547/LConn1 -- Redacted_9896/RConn1
  Redacted_7163/RConn1 -- Redacted_2324/LConn1
  Redacted_3677/RConn1 -- Redacted_8236/LConn1
  Redacted_358/RConn1 -- Redacted_3121/LConn1
  Redacted_5137/LConn1 -- Redacted_4213/RConn1
  Redacted_916/LConn1 -- Redacted_2467/RConn1
  Redacted_2448/RConn1 -- Redacted_9356/LConn1
  Redacted_7498/LConn1 -- Redacted_6556/RConn1
  Redacted_3420/RConn1 -- Redacted_8641/LConn1
  Redacted_8014/LConn1 -- Redacted_9284/RConn1
  Redacted_2433/LConn1 -- Redacted_8330/RConn1
  Redacted_4277/LConn1 -- Redacted_7333/RConn1
  Redacted_5265/RConn1 -- Redacted_323/LConn1
  Redacted_4670/RConn1 -- Redacted_4317/LConn1
  Redacted_4795/RConn1 -- Redacted_1064/RConn1 -- Redacted_2124/LConn1
  Redacted_5313/RConn1 -- Redacted_8644/LConn1 -- Redacted_5467/RConn1
  Redacted_1805/LConn1 -- Redacted_8461/RConn1 -- Redacted_5261/RConn1
  Redacted_7974/RConn1 -- Redacted_7362/RConn1 -- Redacted_6375/LConn1
  Redacted_3355/LConn1 -- Redacted_5541/RConn1 -- Redacted_9821/RConn1
  Redacted_7010/RConn1 -- Redacted_4038/RConn1 -- Redacted_1595/LConn1
  Redacted_9114/LConn1 -- Redacted_7117/RConn1 -- Redacted_5428/RConn1
  Redacted_7456/LConn1 -- Redacted_8468/RConn1 -- Redacted_3035/RConn1

== system Electrical_System_2018b_obfs/Redacted_1750/Redacted_5682 ==
  note: Transient
  note: Steady State
  Redacted_8066 : Subsystem  VariantControl=Choice
  Redacted_9895 : PMIOPort  Side=Left
  Redacted_6360 : PMIOPort  Port=2  Side=Left
  Redacted_7645 : PMIOPort  Port=3  Side=Left
  Redacted_2461 : PMIOPort  Port=4  Side=Left
  Redacted_3445 : PMIOPort  Port=5  Side=Right
  Redacted_5329 : PMIOPort  Port=6  Side=Right
  Redacted_8781 : PMIOPort  Port=7  Side=Right
  Redacted_5062 : PMIOPort  Port=8  Side=Right

== system Electrical_System_2018b_obfs/Redacted_1750/Redacted_7456 ==
  note: Steady State
  note: Transient
  Redacted_986 : Subsystem  VariantControl=Variant1
  Redacted_2977 : PMIOPort  Side=Left
  Redacted_8753 : PMIOPort  Port=2  Side=Left

== system Electrical_System_2018b_obfs/Redacted_1750/Redacted_7650 ==
  note: Transient
  note: Steady State
  Redacted_6349 : Subsystem  VariantControl=Choice
  Redacted_956 : PMIOPort  Side=Left
  Redacted_372 : PMIOPort  Port=2  Side=Left
  Redacted_7777 : PMIOPort  Port=3  Side=Left
  Redacted_2409 : PMIOPort  Port=4  Side=Left
  Redacted_4885 : PMIOPort  Port=5  Side=Left
  Redacted_8935 : PMIOPort  Port=6  Side=Left
  Redacted_4304 : PMIOPort  Port=7  Side=Left
  Redacted_3066 : PMIOPort  Port=8  Side=Left

== system Electrical_System_2018b_obfs/Redacted_1750/Redacted_8299 ==
  note: Transient
  note: Steady State
  Redacted_4710 : Subsystem  VariantControl=Choice
  Redacted_4573 : PMIOPort  Side=Left
  Redacted_1220 : PMIOPort  Port=2  Side=Left
  Redacted_2982 : PMIOPort  Port=3  Side=Left
  Redacted_3513 : PMIOPort  Port=4  Side=Left
  Redacted_6567 : PMIOPort  Port=5  Side=Left
  Redacted_5311 : PMIOPort  Port=6  Side=Left

== system Electrical_System_2018b_obfs/Redacted_1750/Redacted_8712 ==
  note: Steady State
  note: Transient
  Redacted_4950 : Subsystem  VariantControl=Choice
  Redacted_9087 : PMIOPort  Side=Left
  Redacted_8009 : PMIOPort  Port=2  Side=Left
  Redacted_6326 : PMIOPort  Port=3  Side=Left
  Redacted_1150 : PMIOPort  Port=4  Side=Left
  Redacted_6426 : PMIOPort  Port=5  Side=Left
  Redacted_8072 : PMIOPort  Port=6  Side=Left
  Redacted_4470 : PMIOPort  Port=7  Side=Left
  Redacted_1909 : PMIOPort  Port=8  Side=Left
  Redacted_4712 : PMIOPort  Port=9  Side=Left
  Redacted_327 : PMIOPort  Port=10  Side=Left
  Redacted_3395 : PMIOPort  Port=11  Side=Left
  Redacted_6977 : PMIOPort  Port=12  Side=Left
  Redacted_4149 : PMIOPort  Port=13  Side=Left
  Redacted_8379 : PMIOPort  Port=14  Side=Left
  Redacted_6062 : PMIOPort  Port=15  Side=Left
  Redacted_8951 : PMIOPort  Port=16  Side=Left
  Redacted_7229 : PMIOPort  Port=17  Side=Left
  Redacted_3428 : PMIOPort  Port=18  Side=Left
  Redacted_7060 : PMIOPort  Port=19  Side=Left
  Redacted_6164 : PMIOPort  Port=20  Side=Left
  Redacted_8396 : PMIOPort  Port=21  Side=Left
  Redacted_9604 : PMIOPort  Port=22  Side=Left
  Redacted_4313 : PMIOPort  Port=23  Side=Left
  Redacted_8906 : PMIOPort  Port=24  Side=Left
  Redacted_3745 : PMIOPort  Port=25  Side=Left
  Redacted_1444 : PMIOPort  Port=26  Side=Left

== system Electrical_System_2018b_obfs/Redacted_4814/Redacted_3297 ==
  note: Steady State
  note: Transient
  Redacted_8203 : Subsystem  VariantControl=Choice
  Redacted_6460 : PMIOPort  Side=Right
  Redacted_9119 : PMIOPort  Port=2  Side=Right
  Redacted_4230 : PMIOPort  Port=3  Side=Right
  Redacted_901 : PMIOPort  Port=4  Side=Right

== system Electrical_System_2018b_obfs/Redacted_4814/Redacted_3928 ==
  note: Transient
  note: Steady State
  Redacted_4232 : Subsystem  VariantControl=Choice
  Redacted_8727 : PMIOPort  Side=Right
  Redacted_5217 : PMIOPort  Port=2  Side=Right
  Redacted_8285 : PMIOPort  Port=3  Side=Right
  Redacted_9547 : PMIOPort  Port=4  Side=Right

== system Electrical_System_2018b_obfs/Redacted_9930/Redacted_3896 ==
  note: Transient
  note: Steady State
  Redacted_7665 : Subsystem  VariantControl=Variant1
  Redacted_644 : Outport
  Redacted_2723 : Outport  Port=2
  Redacted_8075 : Outport  Port=3
  Redacted_4126 : Outport  Port=4
  Redacted_7964 : Outport  Port=5
  Redacted_8682 : Outport  Port=6
  Redacted_6320 : Outport  Port=7
  Redacted_340 : Outport  Port=8
  Redacted_2756 : Outport  Port=9
  Redacted_3273 : Outport  Port=10
  Redacted_4657 : Outport  Port=11
  Redacted_3395 : Outport  Port=12
  Redacted_9977 : Outport  Port=13
  Redacted_2599 : Outport  Port=14
  Redacted_1407 : Outport  Port=15
  Redacted_9412 : Outport  Port=16
  Redacted_123 : Outport  Port=17
  Redacted_8209 : Outport  Port=18
  Redacted_531 : Outport  Port=19
  Redacted_6389 : Outport  Port=20
  Redacted_6836 : Outport  Port=21
  Redacted_5007 : Outport  Port=22
  Redacted_6497 : Outport  Port=23
  Redacted_9632 : Outport  Port=24
  Redacted_2902 : Outport  Port=25
  Redacted_2695 : Outport  Port=26
  Redacted_8396 : Outport  Port=27
  Redacted_9164 : Outport  Port=28
  Redacted_9075 : Outport  Port=29
  Redacted_6090 : Outport  Port=30

== system Electrical_System_2018b_obfs/Redacted_9930/Redacted_4814 ==
  note: Steady State
  note: Transient
  Redacted_6431 : Subsystem  VariantControl=Variant1
  Redacted_6479 : Outport
  Redacted_3532 : Outport  Port=2
  Redacted_6579 : Outport  Port=3
  Redacted_5091 : Outport  Port=4
  Redacted_5066 : Outport  Port=5
  Redacted_2648 : Outport  Port=6
  Redacted_3799 : Outport  Port=7
  Redacted_988 : Outport  Port=8
  Redacted_4741 : Outport  Port=9
  Redacted_474 : Outport  Port=10
  Redacted_4041 : Outport  Port=11
  Redacted_9998 : Outport  Port=12
  Redacted_2742 : Outport  Port=13
  Redacted_5781 : Outport  Port=14
  Redacted_125 : Outport  Port=15
  Redacted_4308 : Outport  Port=16
  Redacted_8077 : Outport  Port=17
  Redacted_7701 : Outport  Port=18
  Redacted_8967 : Outport  Port=19
  Redacted_8464 : Outport  Port=20
  Redacted_1093 : Outport  Port=21
  Redacted_1950 : Outport  Port=22
  Redacted_1167 : Outport  Port=23
  Redacted_3969 : Outport  Port=24
  Redacted_1905 : Outport  Port=25
  Redacted_1688 : Outport  Port=26
  Redacted_6009 : Outport  Port=27
  Redacted_9612 : Outport  Port=28
  Redacted_8082 : Outport  Port=29
  Redacted_1556 : Outport  Port=30

== system Electrical_System_2018b_obfs/Redacted_1221/Redacted_346/Redacted_2722 ==
  Redacted_6167 : Inport
  Redacted_3224 : SimscapeBus  HierarchyStrings=Redacted_9752;Redacted_8153
  Redacted_5748 : SimscapeBus  HierarchyStrings=Redacted_8561;Redacted_9790;Redacted_365;Redacted_7339;Redacted_2097;Redacted_9030;Redacted_5013;Redacted_897
  Redacted_8690 : SimscapeBus  HierarchyStrings=Redacted_9189;Redacted_9057
  Redacted_9748 : Subsystem  VariantControlMode=Label  Variant=on  VariantControl=Variant1  LabelModeActiveChoice=Variant1
  Redacted_4664 : PMIOPort  Side=Left
  Redacted_1476 : Outport
  wires:
  Redacted_6167/1 -> Redacted_9748/1(Redacted_8203)
  Redacted_9748/1(Redacted_8085) -> Redacted_1476/1
  connections:
  Redacted_9748/LConn5 -- Redacted_5748/LConn6
  Redacted_3224/LConn1 -- Redacted_9748/LConn1
  Redacted_9748/LConn3 -- Redacted_5748/LConn8
  Redacted_5748/LConn2 -- Redacted_9748/RConn2
  Redacted_9748/LConn6 -- Redacted_5748/LConn5
  Redacted_3224/LConn2 -- Redacted_9748/LConn2
  Redacted_9748/LConn4 -- Redacted_5748/LConn7
  Redacted_5748/LConn1 -- Redacted_9748/RConn1
  Redacted_5748/LConn3 -- Redacted_9748/RConn3
  Redacted_9748/RConn4 -- Redacted_5748/LConn4
  Redacted_8690/LConn2 -- Redacted_5748/RConn1
  Redacted_8690/LConn1 -- Redacted_3224/RConn1
  Redacted_8690/RConn1 -- Redacted_4664/RConn1

== system Electrical_System_2018b_obfs/Redacted_1221/Redacted_346/Redacted_3067 ==
  Redacted_882 : Inport
  Redacted_1256 : SimscapeBus  HierarchyStrings=Redacted_9642;Redacted_3041
  Redacted_5519 : Subsystem  VariantControlMode=Label  Variant=on  VariantControl=Variant1  LabelModeActiveChoice=Choice
  Redacted_8046 : SimscapeBus  HierarchyStrings=Redacted_722;Redacted_9678;Redacted_3415
  Redacted_9594 : SimscapeBus  HierarchyStrings=Redacted_8618;Redacted_4044
  Redacted_3488 : PMIOPort  Side=Left
  Redacted_7765 : Outport
  wires:
  Redacted_882/1 -> Redacted_5519/1(Redacted_7936)
  Redacted_5519/1(Redacted_4854) -> Redacted_7765/1
  connections:
  Redacted_8046/LConn1 -- Redacted_5519/RConn1
  Redacted_5519/LConn2 -- Redacted_9594/LConn2
  Redacted_8046/LConn3 -- Redacted_5519/RConn3
  Redacted_5519/LConn1 -- Redacted_9594/LConn1
  Redacted_8046/LConn2 -- Redacted_5519/RConn2
  Redacted_1256/LConn1 -- Redacted_9594/RConn1
  Redacted_1256/LConn2 -- Redacted_8046/RConn1
  Redacted_1256/RConn1 -- Redacted_3488/RConn1

== system Electrical_System_2018b_obfs/Redacted_1221/Redacted_346/Redacted_5295 ==
  Redacted_8545 : Inport
  Redacted_5142 : SimscapeBus  HierarchyStrings=Redacted_8068;Redacted_1994
  Redacted_5826 : SimscapeBus  HierarchyStrings=Redacted_7858;Redacted_5937;Redacted_409;Redacted_2792
  Redacted_6865 : SimscapeBus  HierarchyStrings=Redacted_5281;Redacted_3924;Redacted_7143
  Redacted_8149 : SimscapeBus  HierarchyStrings=Redacted_9603
  Redacted_9050 : SimscapeBus  HierarchyStrings=Redacted_5903
  Redacted_9981 : Subsystem  VariantControlMode=Label  Variant=on  VariantControl=Variant1  LabelModeActiveChoice=Choice
  Redacted_5024 : PMIOPort  Side=Left
  Redacted_7641 : Outport
  wires:
  Redacted_8545/1 -> Redacted_9981/1(Redacted_3927)
  Redacted_9981/1(Redacted_8702) -> Redacted_7641/1
  connections:
  Redacted_5826/RConn1 -- Redacted_5024/RConn1
  Redacted_9981/LConn3 -- Redacted_5142/LConn1
  Redacted_9981/RConn2 -- Redacted_6865/LConn2
  Redacted_9981/LConn1 -- Redacted_8149/LConn1
  Redacted_9981/RConn3 -- Redacted_6865/LConn3
  Redacted_9981/LConn2 -- Redacted_9050/LConn1
  Redacted_9981/RConn1 -- Redacted_6865/LConn1
  Redacted_9981/LConn4 -- Redacted_5142/LConn2
  Redacted_5826/LConn1 -- Redacted_8149/RConn1
  Redacted_5826/LConn2 -- Redacted_9050/RConn1
  Redacted_5826/LConn3 -- Redacted_5142/RConn1
  Redacted_6865/RConn1 -- Redacted_5826/LConn4
